simulink model "UDP_22"  (R2013b)
settings: Solver=ode45  StartTime=0.0  StopTime=1000  MaxStep=0.01  MinStep=0.01  RelTol=1e-3
libraries: dspnetwork x1
settings Model: Creator=lankuohsing  LastModifiedBy=lankuohsing
settings SolverCC: InitialStep=0.01

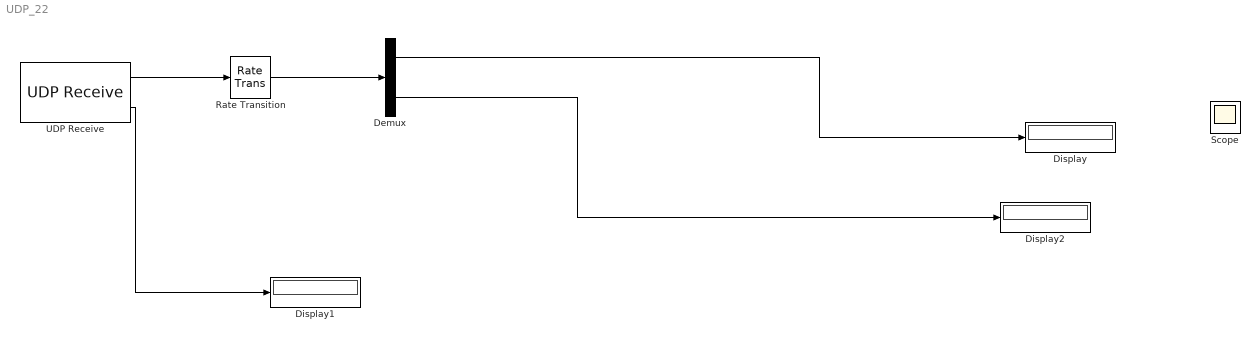
== system UDP_22 ==
  Demux : Demux  Outputs=2
  Display : Display
      settings: Decimation=100
  Display1 : Display
      settings: Decimation=100
  Display2 : Display
      settings: Decimation=100
  Rate Transition : RateTransition  X0=[0 0]  OutPortSampleTime=0.01
  Scope : Scope
  UDP Receive : dspnetwork/UDP Receive  localURL='0.0.0.0'  localPort=9090  remoteURL='0.0.0.0'  remotePort=-1  recvBufferSize=43021  dims=2  signalDatatype=double  isVarSize=off  showBlockingTime=on  blockingTime=inf  sampletime=0.01  blockPlatform=HOST
  wires:
  Demux/1 -> Display/1
  UDP Receive/2 -> Display1/1
  Demux/2 -> Display2/1
  UDP Receive/1 -> Rate Transition/1
  Rate Transition/1 -> Demux/1
